simulink library "Power_Alpha"  (R2013b)
settings: Solver=ode45  StartTime=0.0  StopTime=10.0  RelTol=1e-3
undefined symbols (not defined in the file or in its folder): Power
libraries: simulink x1
settings Model: Creator=mbrauer  LastModifiedBy=mbrauer

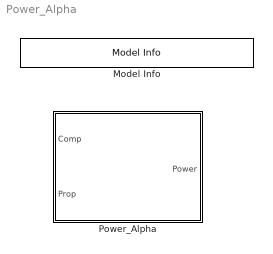
== system Power_Alpha ==
  Model Info : simulink/Model-Wide Utilities/Model Info  InitialBlockCM=None  BlockCM=None  Frame=on  DisplayStringWithTags=Copyright 2013-2014 The MathWorks, Inc.  HorizontalTextAlignment=Center  LeftAlignmentValue=0.5  SourceBlockDiagram=Power_Alpha  TagMaxNumber=20
  Power_Alpha : Subsystem

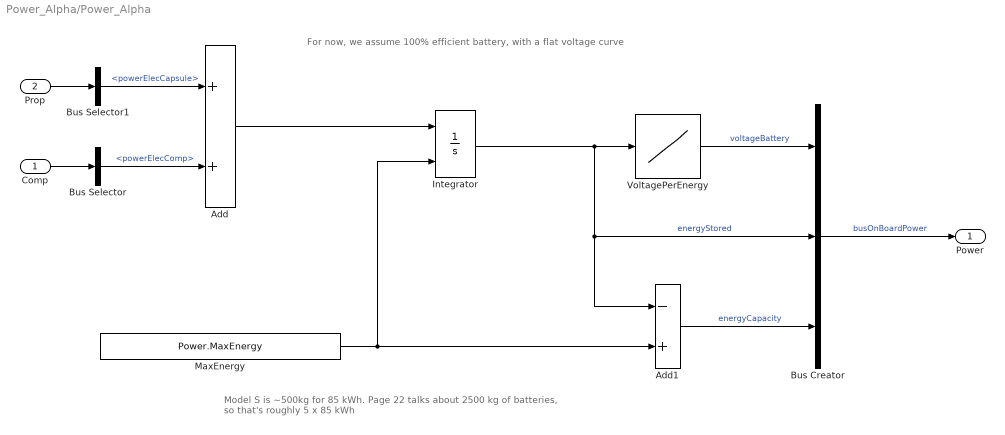
== system Power_Alpha/Power_Alpha ==
  note: Model S is ~500kg for 85 kWh.
      | Page 22 talks about 2500 kg of batteries, so that's roughly 5 x 85 kWh
  note: For now, we assume 100% efficient battery, with a flat voltage curve
  Comp : Inport
  Prop : Inport  Port=2
  Add : Sum
  Add1 : Sum  Inputs=-+
  Bus Creator : BusCreator  Inputs=3  NonVirtualBus=on
  Bus Selector : BusSelector  OutputSignals=powerElecComp
  Bus Selector1 : BusSelector  OutputSignals=powerElecCapsule
  Integrator : Integrator  InitialConditionSource=external
  MaxEnergy : Constant  Value=Power.MaxEnergy
  VoltagePerEnergy : Lookup_n-D  NumberOfTableDimensions=1  BreakpointsForDimension1=[0 1e9]  Table=[600 600]  InternalRulePriority=Speed  RndMeth=Simplest  InputSameDT=on
  Power : Outport
  wires:
  Bus Selector1/1 -> Add/1  "<powerElecCapsule>"
  Integrator/1 -> Add1/1, Bus Creator/2, VoltagePerEnergy/1  "energyStored"
  Bus Creator/1 -> Power/1  "busOnBoardPower"
  Add/1 -> Integrator/1
  MaxEnergy/1 -> Integrator/2, Add1/2
  Bus Selector/1 -> Add/2  "<powerElecComp>"
  Prop/1 -> Bus Selector1/1
  VoltagePerEnergy/1 -> Bus Creator/1  "voltageBattery"
  Add1/1 -> Bus Creator/3  "energyCapacity"
  Comp/1 -> Bus Selector/1
